simulink model "Lab7Simulink"  (R2022b)
settings: Solver=VariableStepAuto  StartTime=0.0  StopTime=czas_symulacji  RelTol=1e-3
values from neighbouring files (symbols this model uses):
  t0 = 500    [lab10.m]
undefined symbols (not defined in the file or in its folder): Cvp, Cvw, dQg, dTzew, Kcp, Kcw, Kcwp, KpIND, KTp, KTp_Styczna, KTwew, KTwew_Styczna, Qg0, T0Tp, T0TpStyczna, T0Twew, T0TwewStyczna, TiIND, Tp0, TTp, TTpStyczna, TTwew, TTwewStyczna, Twew0, Tzew0
settings Model: Creator=Lab320  LastModifiedBy=piter
settings SolverCC: AlgebraicLoopSolver=TrustRegion
settings DataIOCC: ReturnWorkspaceOutputs=off
settings DebuggingCC: UnconnectedInputMsg=warning  UnconnectedOutputMsg=warning  UnconnectedLineMsg=warning  SFMachineParentedDataDiag=warning
settings ModelReferenceCC: EnableRefExpFcnMdlSchedulingChecks=on
settings RTWCC: DLArmComputeVersion=19.05

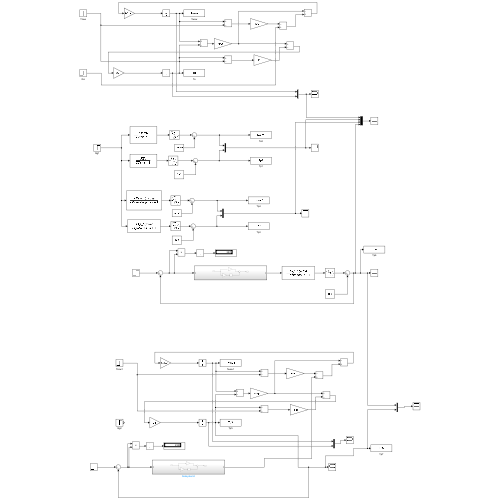
[thumbnail: Simulink's stored preview of the top-level diagram]
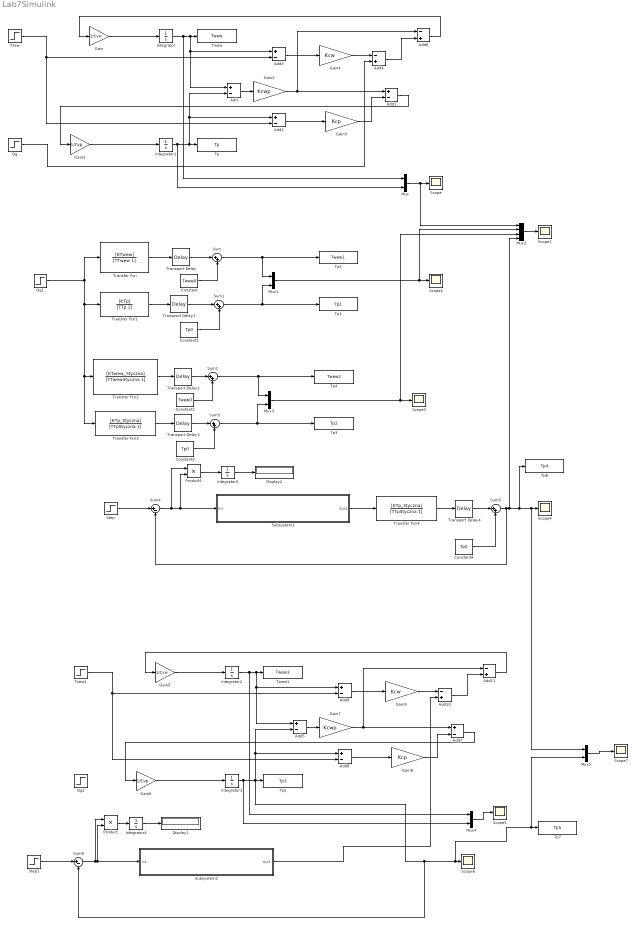
== system Lab7Simulink ==
  Add{,1..3,5,7..9} (8 alike) : Sum  Inputs=+-
  Add{4,6,10..11} (4 alike) : Sum  Inputs=-+
  Constant : Constant  Value=Twew0
  Constant1 : Constant  Value=Tp0
  Constant2 : Constant  Value=Twew0
  Constant3 : Constant  Value=Tp0
  Constant4 : Constant  Value=Tp0
  Display1 : Display
  Display2 : Display
  Gain : Gain  Gain=1/Cvw
  Gain1 : Gain  Gain=1/Cvp
  Gain2 : Gain  Gain=Kcwp
  Gain3 : Gain  Gain=Kcp
  Gain4 : Gain  Gain=Kcw
  Gain5 : Gain  Gain=1/Cvw
  Gain6 : Gain  Gain=1/Cvp
  Gain7 : Gain  Gain=Kcwp
  Gain8 : Gain  Gain=Kcp
  Gain9 : Gain  Gain=Kcw
  Integrator : Integrator  InitialCondition=Twew0
  Integrator1 : Integrator  InitialCondition=Tp0
  Integrator2 : Integrator  InitialCondition=Twew0
  Integrator3 : Integrator  InitialCondition=Tp0
  Integrator4 : Integrator
  Integrator5 : Integrator
  Mux{,1,3..5} (5 alike) : Mux  Inputs=2
  Mux2 : Mux
  Product : Product
  Product1 : Product
  Qg : Step  Time=t0  Before=Qg0  After=Qg0 + dQg  SampleTime=0
  Qg1 : Step  Time=t0  After=dQg  SampleTime=0
  Qg2 : Step  Time=t0  Before=Qg0  After=Qg0 + dQg  SampleTime=0
  Scope{,1..7} (8 alike) : Scope
  Step : Step  Time=t0  Before=Tp0  After=13  SampleTime=0
  Step1 : Step  Time=t0  Before=Tp0  After=13  SampleTime=0
  Subsystem1 : Subsystem
  Subsystem2 : Subsystem
  Sum{,1..3,5} (5 alike) : Sum  Inputs=|++
  Sum4 : Sum  Inputs=|+-
  Sum6 : Sum  Inputs=|+-
  Tp : ToWorkspace  VariableName=Tp  SampleTime=-1
  Tp1 : ToWorkspace  VariableName=Tp1  SampleTime=-1
  Tp2 : ToWorkspace  VariableName=Twew1  SampleTime=-1
  Tp3 : ToWorkspace  VariableName=Tp2  SampleTime=-1
  Tp4 : ToWorkspace  VariableName=Twew2  SampleTime=-1
  Tp5 : ToWorkspace  VariableName=Tp3  SampleTime=-1
  Tp6 : ToWorkspace  VariableName=Tp4  SampleTime=-1
  Tp7 : ToWorkspace  VariableName=Tp5  SampleTime=-1
  Transfer Fcn : TransferFcn  Numerator=[KTwew]  Denominator=[TTwew 1]
  Transfer Fcn1 : TransferFcn  Numerator=[KTp]  Denominator=[TTp 1]
  Transfer Fcn2 : TransferFcn  Numerator=[KTwew_Styczna]  Denominator=[TTwewStyczna 1]
  Transfer Fcn3 : TransferFcn  Numerator=[KTp_Styczna]  Denominator=[TTpStyczna 1]
  Transfer Fcn4 : TransferFcn  Numerator=[KTp_Styczna]  Denominator=[TTpStyczna 1]
  Transport Delay : TransportDelay  DelayTime=T0Twew
  Transport Delay1 : TransportDelay  DelayTime=T0Tp
  Transport Delay2 : TransportDelay  DelayTime=T0TwewStyczna
  Transport Delay3 : TransportDelay  DelayTime=T0TpStyczna
  Transport Delay4 : TransportDelay  DelayTime=T0TpStyczna
  Twew : ToWorkspace  VariableName=Twew  SampleTime=-1
  Twew1 : ToWorkspace  VariableName=Twew3  SampleTime=-1
  Tzew : Step  Time=t0  Before=Tzew0  After=Tzew0 + dTzew  SampleTime=0
  Tzew1 : Step  Time=t0  Before=Tzew0  After=Tzew0 + dTzew  SampleTime=0
  wires:
  Tzew/1 -> Add3/2, Add2/2
  Qg/1 -> Add4/2
  Gain/1 -> Integrator/1
  Gain1/1 -> Integrator1/1
  Integrator/1 -> Mux/1, Add/1, Add3/1, Twew/1
  Integrator1/1 -> Mux/2, Add2/1, Add/2, Tp/1
  Add/1 -> Gain2/1
  Add2/1 -> Gain3/1
  Gain2/1 -> Add6/1, Add1/1
  Gain3/1 -> Add1/2
  Add3/1 -> Gain4/1
  Gain4/1 -> Add4/1
  Add4/1 -> Add6/2
  Add1/1 -> Gain1/1
  Add6/1 -> Gain/1
  Mux/1 -> Mux2/1, Scope/1
  Transfer Fcn1/1 -> Transport Delay1/1
  Transfer Fcn/1 -> Transport Delay/1
  Mux1/1 -> Scope1/1, Mux2/2
  Qg1/1 -> Transfer Fcn1/1, Transfer Fcn3/1, Transfer Fcn2/1, Transfer Fcn/1
  Mux2/1 -> Scope2/1
  Transport Delay1/1 -> Sum1/1
  Transport Delay/1 -> Sum/1
  Constant/1 -> Sum/2
  Sum/1 -> Tp2/1, Mux1/1
  Constant1/1 -> Sum1/2
  Sum1/1 -> Tp1/1, Mux1/2
  Transfer Fcn2/1 -> Transport Delay2/1
  Sum3/1 -> Tp3/1, Mux3/2
  Transfer Fcn3/1 -> Transport Delay3/1
  Sum2/1 -> Tp4/1, Mux3/1
  Constant3/1 -> Sum3/2
  Constant2/1 -> Sum2/2
  Transport Delay2/1 -> Sum2/1
  Transport Delay3/1 -> Sum3/1
  Mux3/1 -> Mux2/3, Scope3/1
  Step/1 -> Sum4/1
  Sum4/1 -> Product1/1, Product1/2, Subsystem1/1(In1)
  Transfer Fcn4/1 -> Transport Delay4/1
  Subsystem1/1(Out1) -> Transfer Fcn4/1
  Transport Delay4/1 -> Sum5/1
  Constant4/1 -> Sum5/2
  Sum5/1 -> Tp6/1, Mux5/1, Scope4/1, Mux2/4, Sum4/2
  Gain8/1 -> Add7/2
  Add5/1 -> Gain7/1
  Add11/1 -> Gain5/1
  Add8/1 -> Gain8/1
  Add10/1 -> Add11/2
  Mux4/1 -> Scope5/1
  Gain7/1 -> Add11/1, Add7/1
  Add9/1 -> Gain9/1
  Integrator2/1 -> Mux4/1, Add5/1, Add9/1, Twew1/1
  Add7/1 -> Gain6/1
  Gain9/1 -> Add10/1
  Gain6/1 -> Integrator3/1
  Gain5/1 -> Integrator2/1
  Tzew1/1 -> Add9/2, Add8/2
  Integrator3/1 -> Mux4/2, Mux5/2, Tp7/1, Scope6/1, Sum6/2, Add8/1, Add5/2, Tp5/1
  Step1/1 -> Sum6/1
  Sum6/1 -> Product/1, Product/2, Subsystem2/1(In1)
  Subsystem2/1(Out1) -> Add10/2
  Mux5/1 -> Scope7/1
  Product/1 -> Integrator4/1
  Product1/1 -> Integrator5/1
  Integrator5/1 -> Display2/1
  Integrator4/1 -> Display1/1

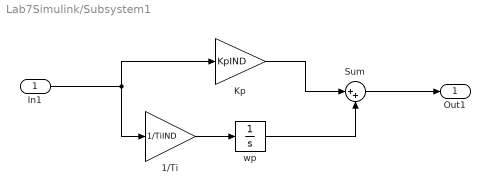
== system Lab7Simulink/Subsystem1 ==
  In1 : Inport
  1/Ti : Gain  Gain=1/TiIND
  Kp : Gain  Gain=KpIND
  Sum : Sum  Inputs=|++
  wp : Integrator
  Out1 : Outport
  wires:
  1/Ti/1 -> wp/1
  In1/1 -> Kp/1, 1/Ti/1
  Kp/1 -> Sum/1
  wp/1 -> Sum/2
  Sum/1 -> Out1/1

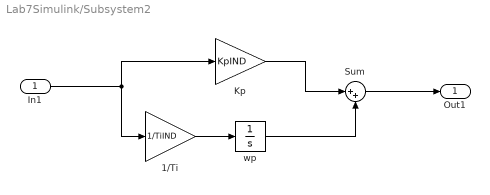
== system Lab7Simulink/Subsystem2 ==
  In1 : Inport
  1/Ti : Gain  Gain=1/TiIND
  Kp : Gain  Gain=KpIND
  Sum : Sum  Inputs=|++
  wp : Integrator  InitialCondition=Qg0
  Out1 : Outport
  wires:
  1/Ti/1 -> wp/1
  In1/1 -> Kp/1, 1/Ti/1
  Kp/1 -> Sum/1
  wp/1 -> Sum/2
  Sum/1 -> Out1/1
